simulink model "C22_basic_queueing_system"  (R2022b)
settings: Solver=VariableStepAuto  StartTime=0.0  StopTime=10.0  RelTol=1e-3
libraries: NSA_DEVS_MATH_OPERATIONS x5, NSA_DEVS_LOGISTICS_QUEUES x4, NSA_DEVS_LOGISTICS_SERVER x4, NSA_DEVS_SINKS x4, NSA_DEVS_ROUTING x3, NSA_DEVS_LOGISTICS_SOURCES x1, NSA_DEVS_LOGISTICS_SINKS x1
settings Model: Creator=david  LastModifiedBy=david

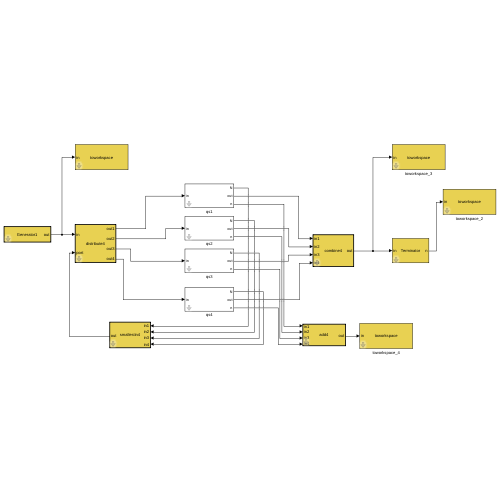
[thumbnail: Simulink's stored preview of the top-level diagram]
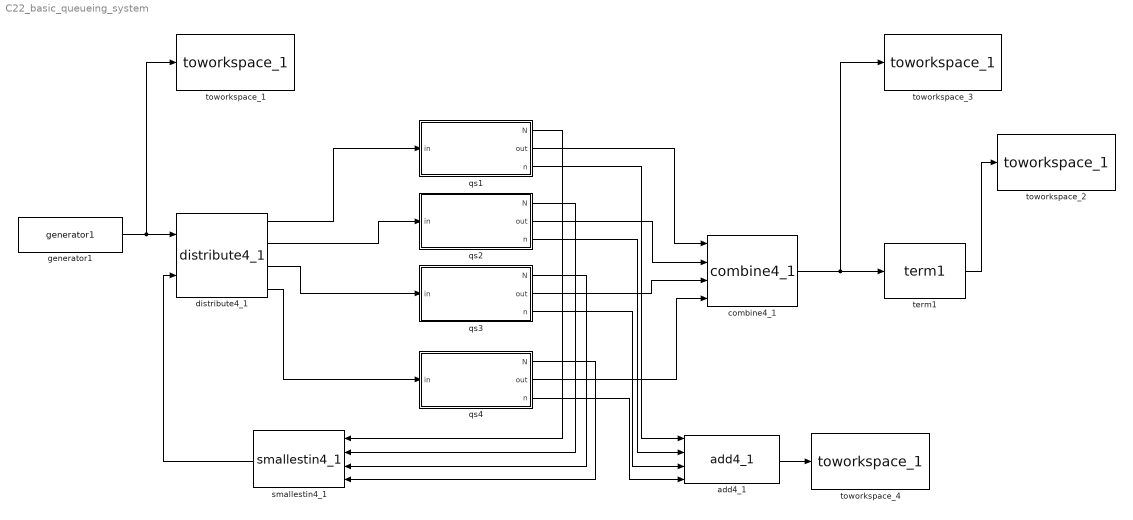
== system C22_basic_queueing_system ==
  add4_1 : NSA_DEVS_MATH_OPERATIONS/add4_1  tau=[0,1]  debug=0  constructor="'add4(\"name\", tau, debug)'"
      settings: SourceProductName=NSA_DEVS
  combine4_1 : NSA_DEVS_ROUTING/combine4_1  tau=[0,5]  debug=0  constructor="'combine4(\"name\", tau, debug)'"
      settings: SourceProductName=NSA_DEVS
  distribute4_1 : NSA_DEVS_ROUTING/distribute4_1  port0=1  tau=[0,20]  debug=0  constructor="'distribute4(\"name\", port0, tau, debug)'"
      settings: SourceProductName=NSA_DEVS
  generator1 : NSA_DEVS_LOGISTICS_SOURCES/generator1  tG=1  n0=1  nG=100  tau=[0,1]  debug=0  constructor="'generator1(\"name\", tG, n0, nG, tau, debug)'"
      settings: SourceProductName=NSA_DEVS
  qs1 : Subsystem  mask{ts=4.5, tau_queue=[0,3]}
  qs2 : Subsystem  mask{ts=4.5, tau_queue=[0,3]}
  qs3 : Subsystem  mask{ts=4.5, tau_queue=[0,3]}
  qs4 : Subsystem  mask{ts=4.5, tau_queue=[0,3]}
  smallestin4_1 : NSA_DEVS_ROUTING/smallestin4_1  tau=[0,1]  debug=0  constructor="'smallestin4(\"name\", tau, debug)'"
      settings: SourceProductName=NSA_DEVS
  term1 : NSA_DEVS_LOGISTICS_SINKS/term1  tau=[0,1]  debug=0  constructor="'terminator(\"name\",tau, debug)'"
      settings: SourceProductName=NSA_DEVS
  toworkspace_1 : NSA_DEVS_SINKS/toworkspace_1  varname="\"'gen_out'\""  t0=0  tau=[0,1]  format="\"'vector'\""  constructor="'toworkspace(\"name\",varname,t0,tau,format)'"
      settings: SourceProductName=NSA_DEVS
  toworkspace_2 : NSA_DEVS_SINKS/toworkspace_1  varname="\"'thrput'\""  t0=0  tau=[0,1]  format="\"'vector'\""  constructor="'toworkspace(\"name\",varname,t0,tau,format)'"
      settings: SourceProductName=NSA_DEVS
  toworkspace_3 : NSA_DEVS_SINKS/toworkspace_1  varname="\"'output'\""  t0=0  tau=[0,1]  format="\"'vector'\""  constructor="'toworkspace(\"name\",varname,t0,tau,format)'"
      settings: SourceProductName=NSA_DEVS
  toworkspace_4 : NSA_DEVS_SINKS/toworkspace_1  varname="\"'SUM_N'\""  t0=0  tau=[0,100]  format="\"'vector'\""  constructor="'toworkspace(\"name\",varname,t0,tau,format)'"
      settings: SourceProductName=NSA_DEVS
  wires:
  generator1/1 -> distribute4_1/1, toworkspace_1/1
  distribute4_1/1 -> qs1/1(in)
  distribute4_1/2 -> qs2/1(in)
  distribute4_1/3 -> qs3/1(in)
  distribute4_1/4 -> qs4/1(in)
  qs1/1(N) -> smallestin4_1/1
  qs2/1(N) -> smallestin4_1/2
  qs3/1(N) -> smallestin4_1/3
  qs4/1(N) -> smallestin4_1/4
  smallestin4_1/1 -> distribute4_1/2
  qs1/2(out) -> combine4_1/1
  qs2/2(out) -> combine4_1/2
  qs3/2(out) -> combine4_1/3
  qs4/2(out) -> combine4_1/4
  combine4_1/1 -> toworkspace_3/1, term1/1
  term1/1 -> toworkspace_2/1
  add4_1/1 -> toworkspace_4/1
  qs1/3(n) -> add4_1/1
  qs2/3(n) -> add4_1/2
  qs3/3(n) -> add4_1/3
  qs4/3(n) -> add4_1/4

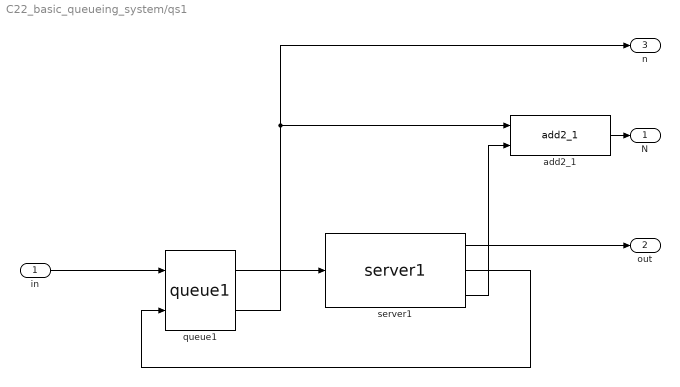
== system C22_basic_queueing_system/qs1 ==
  in : Inport
  add2_1 : NSA_DEVS_MATH_OPERATIONS/add2_1  tau=[0,1]  debug=0  constructor="'add2(\"name\", tau, debug)'"
      settings: SourceProductName=NSA_DEVS
  queue1 : NSA_DEVS_LOGISTICS_QUEUES/queue1  tau=tau_queue  debug=0  tD=tau_queue  constructor="'queue(\"name\", tau, debug, tD)'"
      settings: SourceProductName=NSA_DEVS
  server1 : NSA_DEVS_LOGISTICS_SERVER/server1  ts=ts  tau=[0,1]  debug=0  constructor="'server(\"name\", ts, tau, debug)'"
      settings: SourceProductName=NSA_DEVS
  N : Outport
  out : Outport  Port=2
  n : Outport  Port=3
  wires:
  server1/3 -> add2_1/2
  queue1/2 -> n/1, add2_1/1
  server1/1 -> out/1
  server1/2 -> queue1/2
  add2_1/1 -> N/1
  queue1/1 -> server1/1
  in/1 -> queue1/1

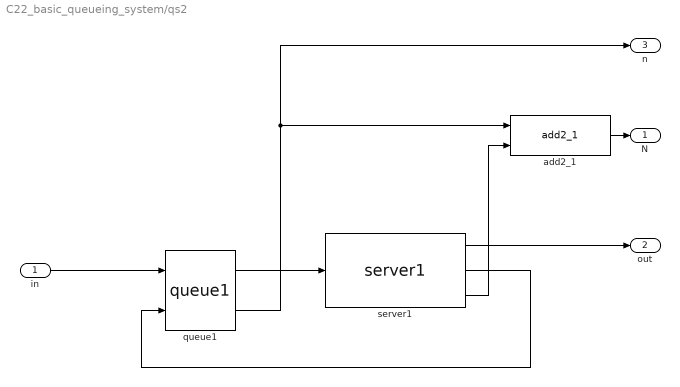
== system C22_basic_queueing_system/qs2 ==
  in : Inport
  add2_1 : NSA_DEVS_MATH_OPERATIONS/add2_1  tau=[0,1]  debug=0  constructor="'add2(\"name\", tau, debug)'"
      settings: SourceProductName=NSA_DEVS
  queue1 : NSA_DEVS_LOGISTICS_QUEUES/queue1  tau=tau_queue  debug=0  tD=tau_queue  constructor="'queue(\"name\", tau, debug, tD)'"
      settings: SourceProductName=NSA_DEVS
  server1 : NSA_DEVS_LOGISTICS_SERVER/server1  ts=ts  tau=[0,1]  debug=0  constructor="'server(\"name\", ts, tau, debug)'"
      settings: SourceProductName=NSA_DEVS
  N : Outport
  out : Outport  Port=2
  n : Outport  Port=3
  wires:
  server1/3 -> add2_1/2
  queue1/2 -> n/1, add2_1/1
  server1/1 -> out/1
  server1/2 -> queue1/2
  add2_1/1 -> N/1
  queue1/1 -> server1/1
  in/1 -> queue1/1

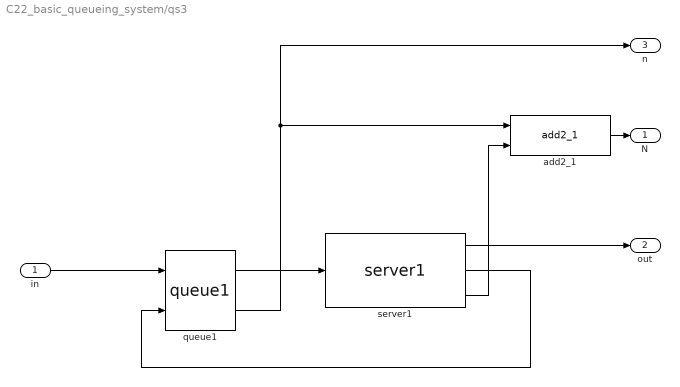
== system C22_basic_queueing_system/qs3 ==
  in : Inport
  add2_1 : NSA_DEVS_MATH_OPERATIONS/add2_1  tau=[0,1]  debug=0  constructor="'add2(\"name\", tau, debug)'"
      settings: SourceProductName=NSA_DEVS
  queue1 : NSA_DEVS_LOGISTICS_QUEUES/queue1  tau=tau_queue  debug=0  tD=tau_queue  constructor="'queue(\"name\", tau, debug, tD)'"
      settings: SourceProductName=NSA_DEVS
  server1 : NSA_DEVS_LOGISTICS_SERVER/server1  ts=ts  tau=[0,1]  debug=0  constructor="'server(\"name\", ts, tau, debug)'"
      settings: SourceProductName=NSA_DEVS
  N : Outport
  out : Outport  Port=2
  n : Outport  Port=3
  wires:
  server1/3 -> add2_1/2
  queue1/2 -> n/1, add2_1/1
  server1/1 -> out/1
  server1/2 -> queue1/2
  add2_1/1 -> N/1
  queue1/1 -> server1/1
  in/1 -> queue1/1

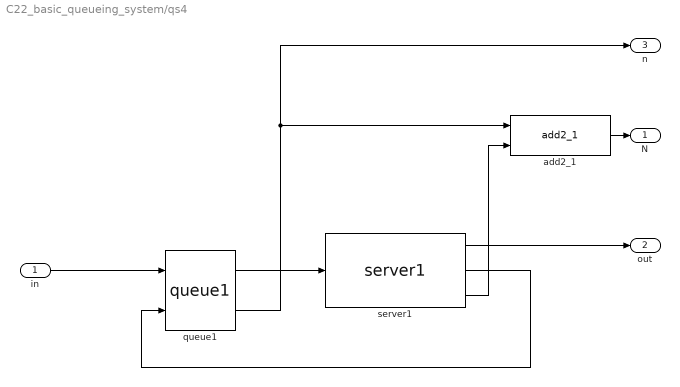
== system C22_basic_queueing_system/qs4 ==
  in : Inport
  add2_1 : NSA_DEVS_MATH_OPERATIONS/add2_1  tau=[0,1]  debug=0  constructor="'add2(\"name\", tau, debug)'"
      settings: SourceProductName=NSA_DEVS
  queue1 : NSA_DEVS_LOGISTICS_QUEUES/queue1  tau=tau_queue  debug=0  tD=tau_queue  constructor="'queue(\"name\", tau, debug, tD)'"
      settings: SourceProductName=NSA_DEVS
  server1 : NSA_DEVS_LOGISTICS_SERVER/server1  ts=ts  tau=[0,1]  debug=0  constructor="'server(\"name\", ts, tau, debug)'"
      settings: SourceProductName=NSA_DEVS
  N : Outport
  out : Outport  Port=2
  n : Outport  Port=3
  wires:
  server1/3 -> add2_1/2
  queue1/2 -> n/1, add2_1/1
  server1/1 -> out/1
  server1/2 -> queue1/2
  add2_1/1 -> N/1
  queue1/1 -> server1/1
  in/1 -> queue1/1
